simulink model "exp5_2"  (Simulink 3.00)
settings: Solver=ode45  StartTime=0.0  StopTime=10.0  RelTol=1e-3

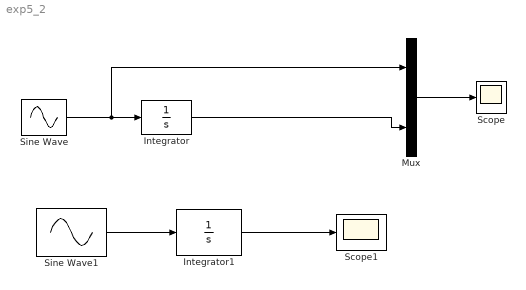
== system exp5_2 ==
  Integrator : Integrator  ExternalReset=none  InitialConditionSource=internal  InitialCondition=0  LimitOutput=off  UpperSaturationLimit=inf  LowerSaturationLimit=-inf  ShowSaturationPort=off  ShowStatePort=off  AbsoluteTolerance=auto
  Integrator1 : Integrator  ExternalReset=none  InitialConditionSource=internal  InitialCondition=0  LimitOutput=off  UpperSaturationLimit=inf  LowerSaturationLimit=-inf  ShowSaturationPort=off  ShowStatePort=off  AbsoluteTolerance=auto
  Mux : Mux  Inputs=2
  Scope : Scope
      settings: TimeRange=10  YMin=-2  YMax=2  SaveToWorkspace=off  SaveName=ScopeData
  Scope1 : Scope
      settings: TimeRange=10  YMin=0  YMax=2  SaveToWorkspace=off  SaveName=ScopeData
  Sine Wave : Sin  Amplitude=[1 2]  Frequency=[1 3]  Phase=0  SampleTime=0
  Sine Wave1 : Sin  Amplitude=1  Frequency=1  Phase=0  SampleTime=0
  wires:
  Integrator/1 -> Mux/2
  Sine Wave/1 -> Integrator/1, Mux/1
  Mux/1 -> Scope/1
  Integrator1/1 -> Scope1/1
  Sine Wave1/1 -> Integrator1/1
